simulink model "servo_simulated"  (R2022a)
settings: Solver=ode45  StartTime=0.0  StopTime=10  RelTol=1e-3  EnableMultiTasking=on
PreLoadFcn:
  | init_servo
values from neighbouring files (symbols this model uses):
  km = 2.95    [define_simulation_process.m]    (also in init_servo.m; servo_model.m)
libraries: cstblocks x3
settings Model: Creator=f96to  LastModifiedBy=jingm
settings SolverCC: AlgebraicLoopSolver=TrustRegion
settings DataIOCC: LimitDataPoints=on  SaveFormat=Array  SignalLoggingSaveFormat=ModelDataLogs  ReturnWorkspaceOutputs=off
settings OptimizationCC: BlockReduction=off  BooleanDataType=off  LifeSpan=inf
settings DebuggingCC: SaveWithParameterizedLinksMsg=none  UnderspecifiedInitializationDetection=Classic  MergeDetectMultiDrivingBlocksExec=none  SignalResolutionControl=TryResolveAllWithWarning  MultiTaskDSMMsg=warning  MultiTaskCondExecSysMsg=none  FcnCallInpInsideContextMsg=warning  UnconnectedInputMsg=warning  UnconnectedOutputMsg=warning  UnconnectedLineMsg=warning  SFUnexpectedBacktrackingDiag=warning  SFNoUnconditionalDefaultTransitionDiag=warning  SFExecutionAtInitializationDiag=none  SFMachineParentedDataDiag=warning  ArithmeticOperatorsInVariantConditions=warning
settings HardwareCC: ProdBitPerSizeT=32  ProdBitPerPtrDiffT=32  ProdWordSize=32  ProdHWDeviceType=Specified  TargetUnknown=on
settings ModelReferenceCC: PropagateSignalLabelsOutOfModel=off
settings SFSimCC: SimUseLocalCustomCode=off  CustomCodeUndefinedFunction=UseInterfaceOnly
settings RTWCC: RTWUseLocalCustomCode=off
settings CodeAppCC: StateflowObjectComments=on
settings GRTTargetCC: TargetLangStandard=C89/C90 (ANSI)  CombineOutputUpdateFcns=off  GRTInterface=on
settings ConfigComp: CovMetricSettings=dw  CovSaveCumulativeToWorkspaceVar=on  CovSaveSingleToWorkspaceVar=on  CovExternalEMLEnable=off

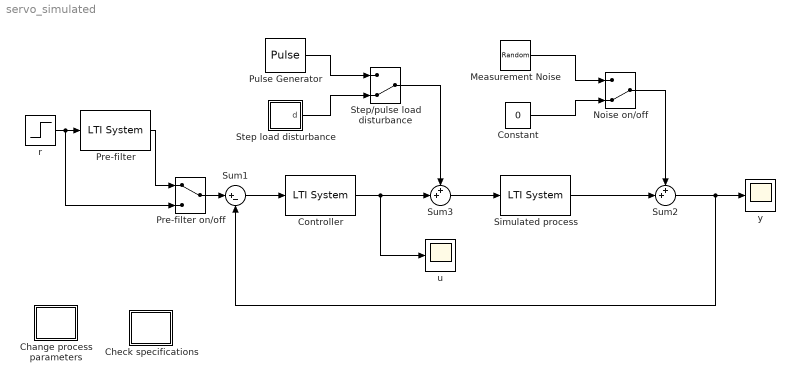
== system servo_simulated ==
  Change process parameters : Subsystem
      settings: OpenFcn=define_simulation_process
  Check specifications : Subsystem
      settings: OpenFcn=specs
  Constant : Constant  Value=0
  Controller : cstblocks/LTI System  sys=C  IC=[]
  Measurement Noise : RandomNumber  Variance=0.05*0.05  Seed=154542  SampleTime=0
  Noise on/off : ManualSwitch  CurrentSetting=0
  Pre-filter : cstblocks/LTI System  sys=F  IC=[]
  "Pre-filter on/off " : ManualSwitch
  Pulse Generator : DiscretePulseGenerator  PulseType=Time based  Amplitude=-1  Period=100  PulseWidth=0.04  PhaseDelay=5
  Simulated process : cstblocks/LTI System  sys=P_sim  IC=[]
  Step load disturbance : Subsystem
  Step/pulse load disturbance : ManualSwitch  CurrentSetting=0
  Sum1 : Sum  Inputs=|+-  InputSameDT=on  SaturateOnIntegerOverflow=on  OutDataTypeStr=Inherit: Same as first input
  Sum2 : Sum  Inputs=++|  InputSameDT=on  SaturateOnIntegerOverflow=on  OutDataTypeStr=Inherit: Same as first input
  Sum3 : Sum  Inputs=++|  InputSameDT=on  SaturateOnIntegerOverflow=on  OutDataTypeStr=Inherit: Same as first input
  r : Step  After=5  SampleTime=0
  u : Scope
  y : Scope
  wires:
  Sum1/1 -> Controller/1
  Controller/1 -> u/1, Sum3/2
  Sum3/1 -> Simulated process/1
  Simulated process/1 -> Sum2/2
  Constant/1 -> Noise on/off/2
  Measurement Noise/1 -> Noise on/off/1
  r/1 -> Pre-filter/1, "Pre-filter on/off "/2
  Step load disturbance/1(d) -> Step/pulse load disturbance/2
  Pulse Generator/1 -> Step/pulse load disturbance/1
  Step/pulse load disturbance/1 -> Sum3/1
  Noise on/off/1 -> Sum2/1
  Sum2/1 -> y/1, Sum1/2
  "Pre-filter on/off "/1 -> Sum1/1
  Pre-filter/1 -> "Pre-filter on/off "/1

== system servo_simulated/Change process parameters ==

== system servo_simulated/Check specifications ==

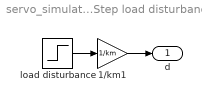
== system servo_simulated/Step load disturbance ==
  1/km1 : Gain  Gain=1/km  SaturateOnIntegerOverflow=on  OutDataTypeStr=Inherit: Same as input  ParamDataTypeStr=Inherit: Same as input
  load disturbance : Step  Time=5  After=-0.15  SampleTime=0
  d : Outport
  wires:
  load disturbance/1 -> 1/km1/1
  1/km1/1 -> d/1
